simulink model "FSTPI"  (R2013a)
settings: Solver=ode45  StartTime=0.0  StopTime=0.2  RelTol=1e-3
libraries: powerlib x25, powerlib_meascontrol x5
settings Model: Creator=DELL  LastModifiedBy=Priti

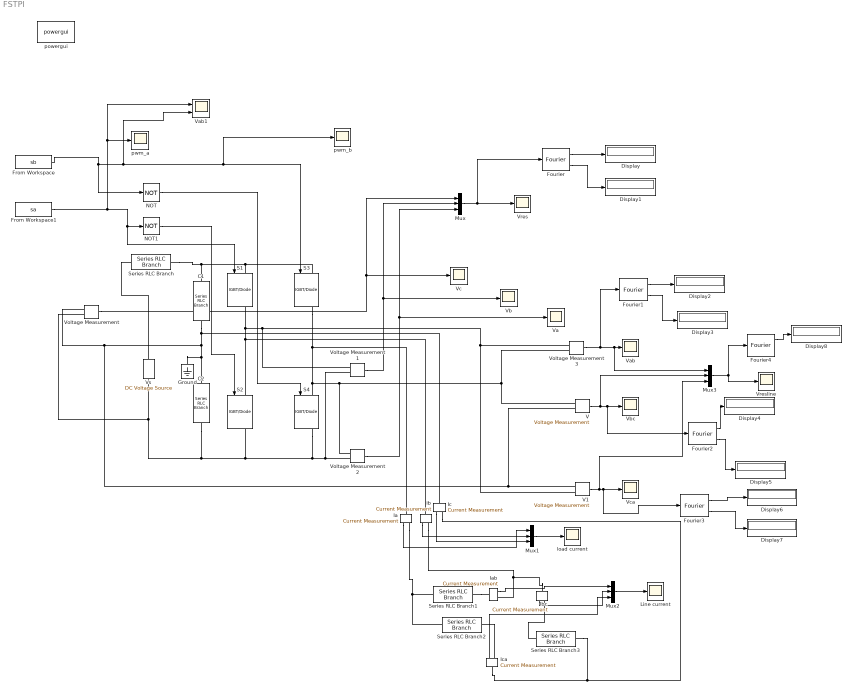
== system FSTPI ==
  C1 : powerlib/Elements/Series RLC Branch  LConnTagsString=__new0  RConnTagsString=__new0  BranchType=C  Resistance=1e-3  Inductance=0  SetiL0=off  InitialCurrent=0  Capacitance=470e-6  Setx0=on  InitialVoltage=50  Measurements=None
  C2 : powerlib/Elements/Series RLC Branch  LConnTagsString=__new0  RConnTagsString=__new0  BranchType=C  Resistance=0  Inductance=0  SetiL0=off  InitialCurrent=0  Capacitance=470e-6  Setx0=on  InitialVoltage=50  Measurements=None
  Display{,1..8} (9 alike) : Display
  Fourier{,1..4} (5 alike) : powerlib_meascontrol/Measurements/Fourier  Freq=50  n=1  InInit=[0, 0]  Ts=0
  From Workspace : FromWorkspace  VariableName=sb  SampleTime=[-1,0]  Interpolate=off  OutputAfterFinalValue=Holding final value
  From Workspace1 : FromWorkspace  VariableName=sa  SampleTime=[-1,0]  Interpolate=off  OutputAfterFinalValue=Setting to zero
  Ground : powerlib/Elements/Ground  LConnTagsString=a
  Ia : powerlib/Measurements/Current Measurement  PhasorSimulation=off  OutputType=Complex  PSBequivalent=0
  Iab : powerlib/Measurements/Current Measurement  PhasorSimulation=off  OutputType=Complex  PSBequivalent=0
  Ibc : powerlib/Measurements/Current Measurement  PhasorSimulation=off  OutputType=Complex  PSBequivalent=0
  Ic : powerlib/Measurements/Current Measurement  PhasorSimulation=off  OutputType=Complex  PSBequivalent=0
  Ica : powerlib/Measurements/Current Measurement  PhasorSimulation=off  OutputType=Complex  PSBequivalent=0
  Line current : Scope
      settings: ShowLegends=on  YMin=-50  YMax=50  SaveName=ScopeData6
  Mux{,1..3} (4 alike) : Mux  Inputs=3
  NOT : Logic  Operator=NOT  AllPortsSameDT=off  OutDataTypeStr=boolean
  NOT1 : Logic  Operator=NOT  AllPortsSameDT=off  OutDataTypeStr=boolean
  S{1..4} (4 alike) : powerlib/Power Electronics/IGBT//Diode  Ron=1e-3  Rs=1e5  Cs=inf  Measurements=on
  Series RLC Branch : powerlib/Elements/Series RLC Branch  LConnTagsString=__new0  RConnTagsString=__new0  BranchType=RL  Resistance=1e-3  Inductance=50e-6  SetiL0=off  InitialCurrent=0  Capacitance=1e-6  Setx0=off  InitialVoltage=0  Measurements=None
  Series RLC Branch1 : powerlib/Elements/Series RLC Branch  LConnTagsString=__new0  RConnTagsString=__new0  BranchType=RL  Resistance=1.405  Inductance=5e-3  SetiL0=off  InitialCurrent=0  Capacitance=1e-6  Setx0=off  InitialVoltage=0  Measurements=None
  Series RLC Branch2 : powerlib/Elements/Series RLC Branch  LConnTagsString=__new0  RConnTagsString=__new0  BranchType=RL  Resistance=1.405  Inductance=5e-3  SetiL0=off  InitialCurrent=0  Capacitance=1e-6  Setx0=off  InitialVoltage=0  Measurements=None
  Series RLC Branch3 : powerlib/Elements/Series RLC Branch  LConnTagsString=__new0  RConnTagsString=__new0  BranchType=RL  Resistance=1.405  Inductance=5e-3  SetiL0=off  InitialCurrent=0  Capacitance=1e-6  Setx0=off  InitialVoltage=0  Measurements=None
  V : powerlib/Measurements/Voltage Measurement  PhasorSimulation=off  OutputType=Complex  PSBequivalent=0
  V1 : powerlib/Measurements/Voltage Measurement  PhasorSimulation=off  OutputType=Complex  PSBequivalent=0
  Va : Scope
      settings: YMin=-400  YMax=400  SaveName=ScopeData5
  Vab : Scope
      settings: YMin=-400  YMax=400  SaveName=ScopeData7
  Vab1 : Scope  NumInputPorts=2
      settings: YMin=-2~-5  YMax=2~5  SaveName=ScopeData12
  Vb : Scope
      settings: YMin=-400  YMax=400  SaveName=ScopeData4
  Vbc : Scope
      settings: YMin=-200  YMax=200  SaveName=ScopeData8
  Vc : Scope
      settings: YMin=-400  YMax=400  SaveName=ScopeData2
  Vca : Scope
      settings: YMin=-200  YMax=200  SaveName=ScopeData9
  Voltage Measurement{,1..3} (4 alike) : powerlib/Measurements/Voltage Measurement  PhasorSimulation=off  OutputType=Complex  PSBequivalent=0
  Vres : Scope
      settings: TimeRange=0.008217324052590874  YMin=-368.9482470784642  YMax=497.4958263772955  SaveName=ScopeData3
  Vresline : Scope
      settings: ShowLegends=on  YMin=-400  YMax=400  SaveName=ScopeData11
  Vs : powerlib/Electrical Sources/DC Voltage Source  Amplitude=100  Measurements=Voltage
  ib : powerlib/Measurements/Current Measurement  PhasorSimulation=off  OutputType=Complex  PSBequivalent=0
  load current : Scope
      settings: ShowLegends=on  SaveName=ScopeData10
  powergui : powerlib/powergui  Priority=1  SimulationMode=Continuous  SolverType=Tustin  SampleTime=50e-6  frequency=60  SPID=off  DisableSnubberDevices=off  DisableRonSwitches=off  DisableVfSwitches=off  SwTol=0  Interpol=off  DisplayEquations=off  frequencyindice=0  Pbase=100e6  ErrMax=1e-4  Iterations=50  UnitsV=kV  UnitsW=MW  FunctionMessages=off  echomessages=off  HookPort=off  EnableUseOfTLC=off  x0status=blocks  RestoreLinks=warning  ResistiveCurrentMeasurement=off  Frange=[0:2:500]  Ylog=off  Xlog=on  ShowGrid=off  save=off  variable=ZData  ZoomFFT=off  StartTime=0.0  cycles=1  DisplayStyle=1  fundamental=60  FreqAxis=off  MaxFrequency=1000  frequencyindicesteady=1  RmsSteady=1  display=off  Ts=0  methode=off
  pwm_a : Scope
      settings: YMin=-20  YMax=20
  pwm_b : Scope
      settings: TimeRange=0.002560000000000001  YMin=-2  YMax=2
  wires:
  Voltage Measurement/1 -> Mux/1, Vc/1
  Voltage Measurement1/1 -> Vb/1, Mux/2
  Voltage Measurement2/1 -> Va/1, Mux/3
  Mux/1 -> Fourier/1, Vres/1
  Fourier/1 -> Display/1
  Fourier/2 -> Display1/1
  NOT1/1 -> S2/1
  From Workspace1/1 -> Vab1/1, pwm_a/1, NOT1/1, S1/1
  NOT/1 -> S4/1
  From Workspace/1 -> NOT/1, S3/1, pwm_b/1, Vab1/2
  Voltage Measurement3/1 -> Fourier1/1, Mux3/1, Vab/1
  V/1 -> Mux3/2, Fourier2/1, Vbc/1
  V1/1 -> Mux3/3, Fourier3/1, Vca/1
  Fourier1/1 -> Display2/1
  Fourier1/2 -> Display3/1
  Fourier2/1 -> Display4/1
  Fourier2/2 -> Display5/1
  Fourier3/1 -> Display6/1
  Fourier3/2 -> Display7/1
  Ia/1 -> Mux1/1
  ib/1 -> Mux1/2
  Ic/1 -> Mux1/3
  Mux1/1 -> load current/1
  Iab/1 -> Mux2/1
  Ibc/1 -> Mux2/2
  Ica/1 -> Mux2/3
  Mux2/1 -> Line current/1
  Mux3/1 -> Vresline/1, Fourier4/1
  Fourier4/1 -> Display8/1
  connections:
  S3/LConn1 -- Series RLC Branch/RConn1 -- C1/LConn1 -- S1/LConn1
  S3/RConn1 -- Ia/LConn1 -- V/LConn1 -- Voltage Measurement3/LConn2 -- Voltage Measurement2/LConn1 -- S4/LConn1
  S4/RConn1 -- Voltage Measurement2/LConn2 -- Voltage Measurement1/LConn2 -- Vs/LConn1 -- Voltage Measurement/LConn2 -- C2/RConn1 -- S2/RConn1
  S2/LConn1 -- ib/LConn1 -- V1/LConn2 -- Voltage Measurement3/LConn1 -- Voltage Measurement1/LConn1 -- S1/RConn1
  V1/LConn1 -- V/LConn2 -- Voltage Measurement/LConn1 -- Ground/LConn1 -- C2/LConn1 -- Ic/LConn1 -- C1/RConn1
  Vs/RConn1 -- Series RLC Branch/LConn1
  ib/RConn1 -- Ibc/LConn1 -- Iab/RConn1
  Ic/RConn1 -- Ica/LConn1 -- Series RLC Branch3/RConn1
  Ia/RConn1 -- Series RLC Branch2/LConn1 -- Series RLC Branch1/LConn1
  Series RLC Branch1/RConn1 -- Iab/LConn1
  Series RLC Branch3/LConn1 -- Ibc/RConn1
  Series RLC Branch2/RConn1 -- Ica/RConn1
